simulink model "DC_motor_state_feedback_control"  (R2024a)
settings: Solver=VariableStepAuto  StartTime=0.0  StopTime=5  MaxStep=0.01  RelTol=1e-3
values from neighbouring files (symbols this model uses):
  b = 0.0000095    (= 9.5e-06)    [init.m]
  J = 0.5*m*r^2    (= 0.000125)    [init.m]
  K = place(Aa, Ba, [-15 -16 -17 -18])    [init.m]
  Kaw = 0    [init.m]
  ke = 0.0191    [init.m]
  kt = 0.0187    [init.m]
  L = 0.35/1000    (= 0.00035)    [init.m]
  R = 0.6    [init.m]
  stp = 15*pi    (= 47.1238898038)    [compare_aw_vs_non_aw.m]    (also in init.m = 3.14159265359)
  tSamp = 0.001    [init.m]
  v_max = 3.5    [compare_aw_vs_non_aw.m]    (also in init.m = inf)
undefined symbols (not defined in the file or in its folder): DiscIntNeverNeededParam
settings Model: Creator=berto  LastModifiedBy=berto

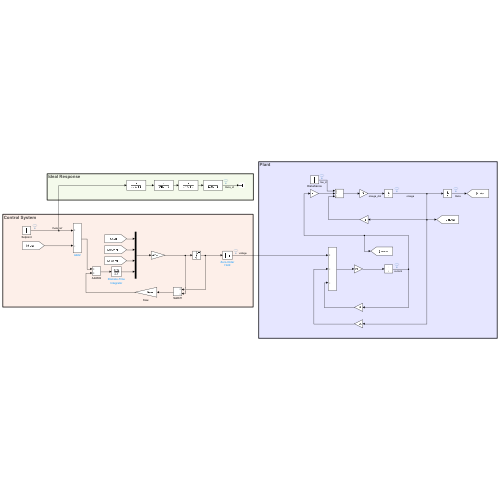
[thumbnail: Simulink's stored preview of the top-level diagram]
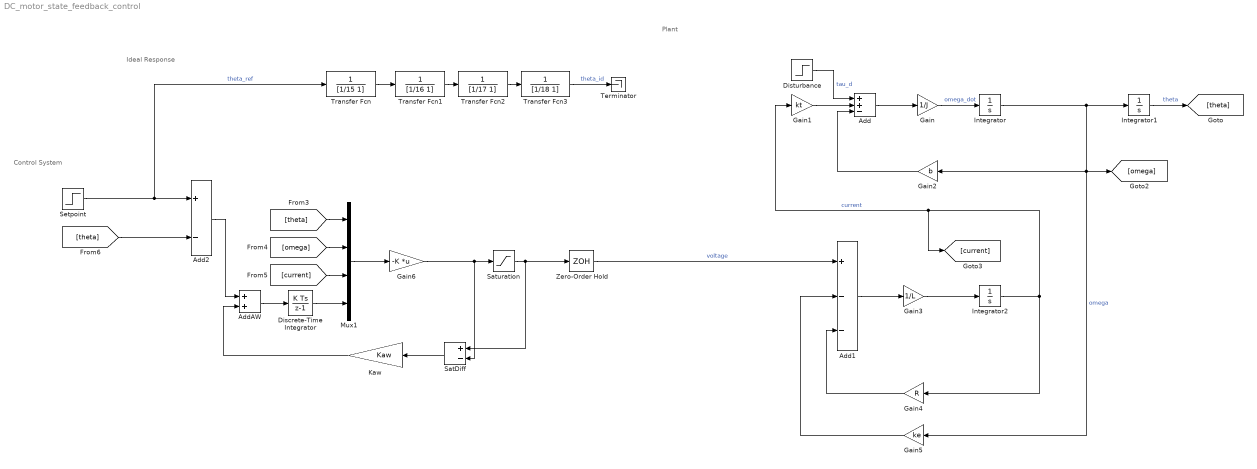
== system DC_motor_state_feedback_control ==
  note: Ideal Response
  note: Control System
  note: Plant
  Add : Sum  Inputs=++-
  Add1 : Sum  Inputs=+--
  Add2 : Sum  Inputs=+-
  AddAW : Sum
  Discrete-Time Integrator : DiscreteIntegrator  SampleTime=tSamp  ICPrevOutput=DiscIntNeverNeededParam  ICPrevScaledInput=DiscIntNeverNeededParam
  Disturbance : Step  Time=2.5  After=0.1  SampleTime=0
  Gain : Gain  Gain=1/J
  Gain1 : Gain  Gain=kt
  Gain2 : Gain  Gain=b
  Gain3 : Gain  Gain=1/L
  Gain4 : Gain  Gain=R
  Gain5 : Gain  Gain=ke
  Gain6 : Gain  Gain=-K  Multiplication=Matrix(K*u)
  Integrator : Integrator
  Integrator1 : Integrator
  Integrator2 : Integrator
  Kaw : Gain  Gain=Kaw
  Mux1 : Mux
  SatDiff : Sum  Inputs=+-
  Saturation : Saturate  UpperLimit=v_max  LowerLimit=-v_max
  Setpoint : Step  After=stp  SampleTime=0
  Terminator : Terminator
  Transfer Fcn : TransferFcn  Denominator=[1/15 1]
  Transfer Fcn1 : TransferFcn  Denominator=[1/16 1]
  Transfer Fcn2 : TransferFcn  Denominator=[1/17 1]
  Transfer Fcn3 : TransferFcn  Denominator=[1/18 1]
  Zero-Order Hold : ZeroOrderHold  SampleTime=tSamp
  wires:
  Integrator/1 -> [omega], Gain2/1, Gain5/1, Integrator1/1  "omega"
  Gain/1 -> Integrator/1  "omega_dot"
  Add/1 -> Gain/1
  Gain1/1 -> Add/2
  Integrator1/1 -> [theta]  "theta"
  Gain2/1 -> Add/3
  Add1/1 -> Gain3/1
  Gain3/1 -> Integrator2/1
  Integrator2/1 -> Gain4/1, [current], Gain1/1  "current"
  Gain4/1 -> Add1/3
  Gain5/1 -> Add1/2
  [theta] -> Mux1/1
  [omega] -> Mux1/2
  [current] -> Mux1/3
  Zero-Order Hold/1 -> Add1/1  "voltage"
  Disturbance/1 -> Add/1  "tau_d"
  Transfer Fcn/1 -> Transfer Fcn1/1
  Transfer Fcn1/1 -> Transfer Fcn2/1
  Transfer Fcn2/1 -> Transfer Fcn3/1
  Transfer Fcn3/1 -> Terminator/1  "theta_id"
  Saturation/1 -> Zero-Order Hold/1, SatDiff/1
  Discrete-Time Integrator/1 -> Mux1/4
  Mux1/1 -> Gain6/1
  [theta] -> Add2/2
  Setpoint/1 -> Add2/1, Transfer Fcn/1  "theta_ref"
  Gain6/1 -> Saturation/1, SatDiff/2
  Add2/1 -> AddAW/1
  Kaw/1 -> AddAW/2
  AddAW/1 -> Discrete-Time Integrator/1
  SatDiff/1 -> Kaw/1
